simulink model "Statechart_Decomposition"  (R2025b)
settings: Solver=FixedStepDiscrete  StartTime=0.0  StopTime=10.0  FixedStep=0.01  RelTol=1e-3
libraries: simulink x1
settings Model: Creator=soura  LastModifiedBy=soura

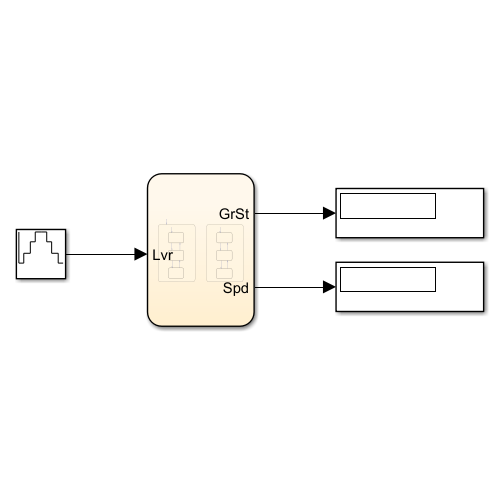
[thumbnail: Simulink's stored preview of the top-level diagram]
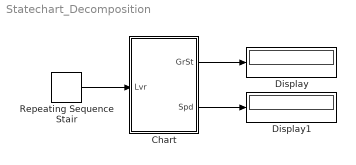
== system Statechart_Decomposition ==
  Chart : Stateflow chart  TreatAsAtomicUnit=on
  Display : Display
  Display1 : Display
  Repeating Sequence Stair : simulink/Sources/Repeating Sequence Stair  OutValues=[1 2 3 4 4 3 2 1].'  tsamp=-1  OutMin=[]  OutMax=[]  OutDataTypeStr=double  OutputDataTypeScalingMode=double  OutDataType=fixdt(0,8)  ConRadixGroup=Best Precision: Vector-wise  OutScaling=2^-12
  wires:
  Repeating Sequence Stair/1 -> Chart/1(Lvr)
  Chart/1(GrSt) -> Display/1
  Chart/2(Spd) -> Display1/1

== stateflow chart Statechart_Decomposition/Chart ==
  state GSL [parallel]
    settings: executionOrder=1
    state Park
      en:GrSt=1;
    state Drive
      en:GrSt=2;
    state Reverse
      en:GrSt=3;
    (default) -> GSL.Park
    GSL.Park -> GSL.Drive : [Lvr==2]
    GSL.Drive -> GSL.Park [order 2] : [Lvr==1]
    GSL.Drive -> GSL.Reverse [order 1] : [Lvr==3]
    GSL.Reverse -> GSL.Drive : [Lvr==2]
  state Display [parallel]
    settings: executionOrder=2
    state Park
      en:Spd=0;
    state Drive
      en:Spd=10;
    state Reverse
      en:Spd=-10;
    (default) -> Display.Park
    Display.Park -> Display.Drive : [Lvr==2]
    Display.Drive -> Display.Park [order 2] : [Lvr==1]
    Display.Drive -> Display.Reverse [order 1] : [Lvr==3]
    Display.Reverse -> Display.Drive : [Lvr==2]
  (default) -> GSL
  data: Lvr input; GrSt output; Spd output
